simulink model "equal_area_piston_sfctrl"  (R2020a)
settings: Solver=ode23tb  StartTime=0.0  StopTime=400  MaxStep=tsample  RelTol=tsample
values from neighbouring files (symbols this model uses):
  A = [0 1; 0 0]    [control_design.m]
  B = [0 1]'    [control_design.m]
  C = [k 0]    [control_design.m]
  K = acker(A,B,poles)    [control_design.m]
  L = acker(A',C',pole_so)'    [control_design.m]
  N = -1/(C*inv(A-B*K)*B)    [control_design.m]
undefined symbols (not defined in the file or in its folder): uc_mac
libraries: fl_lib x21, nesl_utility x20, engine_speed_ctrl_lib x1, engine_OM471_lib x1, load_sensing_pump_lib x1, hydrostatic_fourway_valve_bichamber_piston_lib x1, pm_linear_actuator_lib x1
settings Model: Creator=dbagn  LastModifiedBy=dbagn
settings SolverCC: ZeroCrossControl=DisableAll
settings DataIOCC: SaveTime=off  ReturnWorkspaceOutputs=off

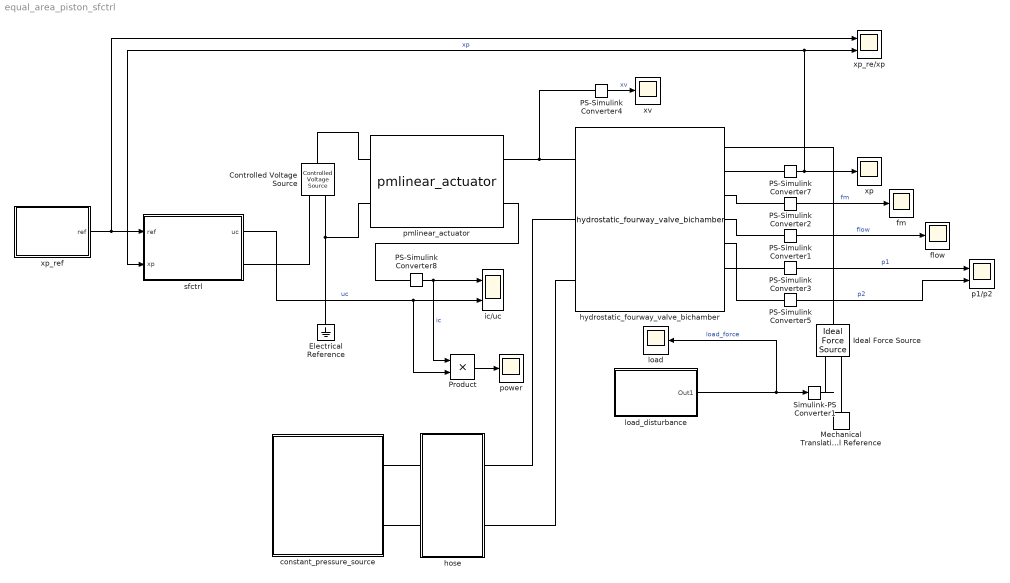
== system equal_area_piston_sfctrl ==
  Controlled Voltage Source : fl_lib/Electrical/Electrical Sources/Controlled Voltage Source
  Electrical Reference : fl_lib/Electrical/Electrical Elements/Electrical Reference
  Ideal Force Source : fl_lib/Mechanical/Mechanical Sources/Ideal Force Source
  Mechanical Translational Reference : fl_lib/Mechanical/Translational Elements/Mechanical Translational Reference
  PS-Simulink Converter{1..5,7..8} (7 alike) : nesl_utility/PS-Simulink Converter  PhysicalDomain=network_engine_domain  SubClassName=ps_output  LeftPortType=input  RightPortType=output  PseudoPeriodic=off  Frequencies=[]  Unit=inherit  AffineConversion=off
  Product : Product
  Simulink-PS Converter1 : nesl_utility/Simulink-PS Converter  PhysicalDomain=network_engine_domain  SubClassName=ps_input  LeftPortType=input  RightPortType=output  PseudoPeriodic=off  Frequencies=[]  NoiseDistribution=none  NoiseParameters=[]  Unit=N  AffineConversion=off  FilteringAndDerivatives=provide  SimscapeFilterOrder=1  InputFilterTimeConstant=0.001  UdotUserProvided=0
  constant_pressure_source : Subsystem
  flow : Scope
  fm : Scope
  hose : Subsystem
  hydrostatic_fourway_valve_bichamber : hydrostatic_fourway_valve_bichamber_piston_lib/hydrostatic_fourway_valve_bichamber  bulk=1.2e9 Pa  rho=850 kg/m^3  D1=0.1 m  D2=0.1 m  Lp=1 m  xv_max=2.75 mm  mp=25 kg  kp=1e5 N/m  bp=2e2 N/(m/s)  q1_specify=off  q1_priority=None  q1=0 m^3/s  q1_nominal_specify=off  q1_nominal_unit=m^3/s  q1_nominal_value=1  q2_specify=off  q2_priority=None  q2=0 m^3/s  q2_nominal_specify=off  q2_nominal_unit=m^3/s  q2_nominal_value=1  qin_specify=off  qin_priority=None  qin=0 m^3/s  qin_nominal_specify=off  qin_nominal_unit=m^3/s  qin_nominal_value=1  qout_specify=off  qout_priority=None  qout=0 m^3/s  qout_nominal_specify=off  qout_nominal_unit=m^3/s  qout_nominal_value=1  p1_specify=off  p1_priority=High  p1=25 bar  p1_nominal_specify=off  p1_nominal_unit=bar  p1_nominal_value=1  p2_specify=off  p2_priority=High  p2=25 bar  p2_nominal_specify=off  p2_nominal_unit=bar  p2_nominal_value=1  fp_specify=off  fp_priority=None  fp=0 N  fp_nominal_specify=off  fp_nominal_unit=N  fp_nominal_value=1  vp_specify=off  vp_priority=None  vp=0 m/s  vp_nominal_specify=off  vp_nominal_unit=m/s  vp_nominal_value=1  xp_specify=off  xp_priority=High  xp=500 mm  xp_nominal_specify=off  xp_nominal_unit=mm  xp_nominal_value=1
      settings: InternalSimscapePortConfiguration="{\"Bottom\":[],\"Left\":[{\"id\":\"xv\",\"label\":\"xv\",\"type\":\"input\"},{\"id\":\"S\",\"label\":\"S\",\"type\":\"foundation.hydraulic.hydraulic\"},{\"id\":\"T\",\"label\":\"T\",\"type\":\"foundation.hydraulic.hydraulic\"}],\"Right\":[{\"id\":\"P\",\"label\":\"P\",\"type\":\"foundation.mechanical.translational.translational\"},{\"id\":\"xp_out\",\"label\":\"xp\",\"type\":\"output\"},{\"id\":\"mforce\",\"label\":\"fm\",\"type\":\"output\"},{\"id\":\"q1_out\",\"label\":\"q1\",\"type\":\"output\"},{\"id\":\"q2_out\",\"label\":\"q2\",\"type\":\"output\"},{\"id\":\"p1_out\",\"label\":\"p1\",\"type\":\"output\"},{\"id\":\"p2_out\",\"label\":\"p2\",\"type\":\"output\"}],\"Top\":[]}"
  ic/uc : Scope  NumInputPorts=2
  load : Scope
  load_disturbance : Subsystem
  p1/p2 : Scope  NumInputPorts=2
  pmlinear_actuator : pm_linear_actuator_lib/pmlinear_actuator  Bm=1 s*V/m^2  mv=0.05 kg  Lc=0.01 H  Rc=10 Ohm  bv=2000 N/(m/s)  h=0.05 m  xv_max=2.75 mm  n=1000  uc_specify=off  uc_priority=None  uc=0 V  uc_nominal_specify=off  uc_nominal_unit=V  uc_nominal_value=1  ic_specify=off  ic_priority=High  ic=0 A  ic_nominal_specify=off  ic_nominal_unit=A  ic_nominal_value=1  vv_specify=off  vv_priority=None  vv=0 m/s  vv_nominal_specify=off  vv_nominal_unit=m/s  vv_nominal_value=1  xv_specify=off  xv_priority=None  xv=0 m  xv_nominal_specify=off  xv_nominal_unit=m  xv_nominal_value=1
      settings: InternalSimscapePortConfiguration="{\"Bottom\":[],\"Left\":[{\"id\":\"ucp\",\"label\":\"ucp\",\"type\":\"foundation.electrical.electrical\"},{\"id\":\"ucn\",\"label\":\"ucn\",\"type\":\"foundation.electrical.electrical\"}],\"Right\":[{\"id\":\"xv_out\",\"label\":\"xv\",\"type\":\"output\"},{\"id\":\"ic_out\",\"label\":\"ic\",\"type\":\"output\"}],\"Top\":[]}"
  power : Scope
  sfctrl : Subsystem
  xp : Scope
  xp_re/xp : Scope  NumInputPorts=2
  xp_ref : Subsystem
  xv : Scope
  wires:
  load_disturbance/1(Out1) -> load/1, Simulink-PS Converter1/1  "load_force"
  PS-Simulink Converter7/1 -> xp_re/xp/2, sfctrl/2(xp), xp/1  "xp"
  PS-Simulink Converter1/1 -> flow/1  "flow"
  PS-Simulink Converter2/1 -> fm/1  "fm"
  PS-Simulink Converter3/1 -> p1/p2/1  "p1"
  xp_ref/1(ref) -> xp_re/xp/1, sfctrl/1(ref)
  PS-Simulink Converter5/1 -> p1/p2/2  "p2"
  PS-Simulink Converter8/1 -> Product/1, ic/uc/1  "ic"
  sfctrl/1("uc ") -> Product/2, ic/uc/2  "uc"
  Product/1 -> power/1
  PS-Simulink Converter4/1 -> xv/1  "xv"
  connections:
  Mechanical Translational Reference/LConn1 -- Ideal Force Source/RConn2
  Simulink-PS Converter1/RConn1 -- Ideal Force Source/RConn1
  constant_pressure_source/RConn1 -- hose/LConn1
  constant_pressure_source/RConn2 -- hose/LConn2
  hydrostatic_fourway_valve_bichamber/LConn2 -- hose/RConn1
  hydrostatic_fourway_valve_bichamber/LConn3 -- hose/RConn2
  hydrostatic_fourway_valve_bichamber/RConn4 -- PS-Simulink Converter1/LConn1
  hydrostatic_fourway_valve_bichamber/RConn3 -- PS-Simulink Converter2/LConn1
  hydrostatic_fourway_valve_bichamber/RConn2 -- PS-Simulink Converter7/LConn1
  hydrostatic_fourway_valve_bichamber/RConn1 -- Ideal Force Source/LConn1
  hydrostatic_fourway_valve_bichamber/RConn5 -- PS-Simulink Converter3/LConn1
  hydrostatic_fourway_valve_bichamber/RConn6 -- PS-Simulink Converter5/LConn1
  Electrical Reference/LConn1 -- pmlinear_actuator/LConn2 -- Controlled Voltage Source/RConn2
  pmlinear_actuator/LConn1 -- Controlled Voltage Source/LConn1
  pmlinear_actuator/RConn1 -- PS-Simulink Converter4/LConn1 -- hydrostatic_fourway_valve_bichamber/LConn1
  pmlinear_actuator/RConn2 -- PS-Simulink Converter8/LConn1
  sfctrl/RConn1 -- Controlled Voltage Source/RConn1

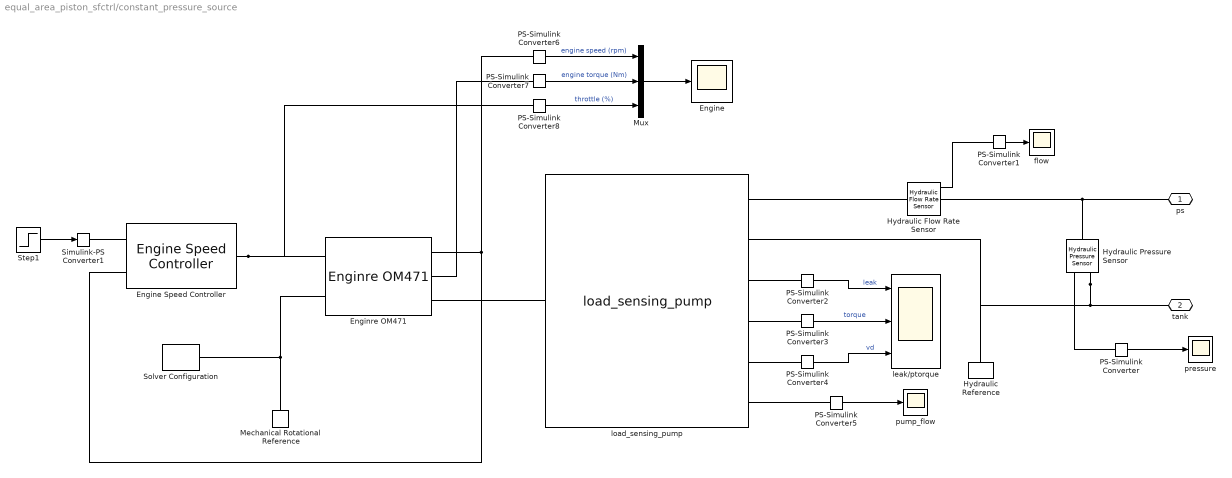
== system equal_area_piston_sfctrl/constant_pressure_source ==
  Engine : Scope
  Engine Speed Controller : engine_speed_ctrl_lib/Engine Speed Controller  kp=1e-3/2 s  kint=1e-2/2  kd=0 s^2  t_out_specify=off  t_out_priority=High  t_out=0  t_out_nominal_specify=off  t_out_nominal_unit=1  t_out_nominal_value=1
      settings: InternalSimscapePortConfiguration="{\"Bottom\":[],\"Left\":[{\"id\":\"we_ref\",\"label\":\"we_ref\",\"type\":\"input\"},{\"id\":\"we\",\"label\":\"we\",\"type\":\"input\"}],\"Right\":[{\"id\":\"theta\",\"label\":\"theta\",\"type\":\"output\"}],\"Top\":[]}"
  Enginre OM471 : engine_OM471_lib/Enginre OM471  dynamic_responce=simscape.enum.onoff.on  cshaft_inertia=5 kg*m^2  initial_speed=800
      settings: InternalSimscapePortConfiguration="{\"Bottom\":[],\"Left\":[{\"id\":\"theta\",\"label\":\"theta\",\"type\":\"input\"},{\"id\":\"C\",\"label\":\"C\",\"type\":\"foundation.mechanical.rotational.rotational\"}],\"Right\":[{\"id\":\"we\",\"label\":\"we\",\"type\":\"output\"},{\"id\":\"te\",\"label\":\"te\",\"type\":\"output\"},{\"id\":\"D\",\"label\":\"D\",\"type\":\"foundation.mechanical.rotational.rotational\"}],\"Top\":[]}"
  Hydraulic Flow Rate Sensor : fl_lib/Hydraulic/Hydraulic Sensors/Hydraulic Flow Rate Sensor
  Hydraulic Pressure Sensor : fl_lib/Hydraulic/Hydraulic Sensors/Hydraulic Pressure Sensor
  Hydraulic Reference : fl_lib/Hydraulic/Hydraulic Elements/Hydraulic Reference
  Mechanical Rotational Reference : fl_lib/Mechanical/Rotational Elements/Mechanical Rotational Reference
  Mux : Mux  Inputs=3
  PS-Simulink Converter : nesl_utility/PS-Simulink Converter  PhysicalDomain=network_engine_domain  SubClassName=ps_output  LeftPortType=input  RightPortType=output  PseudoPeriodic=off  Frequencies=[]  Unit=bar  AffineConversion=on
  PS-Simulink Converter1 : nesl_utility/PS-Simulink Converter  PhysicalDomain=network_engine_domain  SubClassName=ps_output  LeftPortType=input  RightPortType=output  PseudoPeriodic=off  Frequencies=[]  Unit=l/min  AffineConversion=on
  PS-Simulink Converter{2..5} (4 alike) : nesl_utility/PS-Simulink Converter  PhysicalDomain=network_engine_domain  SubClassName=ps_output  LeftPortType=input  RightPortType=output  PseudoPeriodic=off  Frequencies=[]  Unit=1  AffineConversion=off
  PS-Simulink Converter6 : nesl_utility/PS-Simulink Converter  PhysicalDomain=network_engine_domain  SubClassName=ps_output  LeftPortType=input  RightPortType=output  PseudoPeriodic=off  Frequencies=[]  Unit=inherit  AffineConversion=off
  PS-Simulink Converter7 : nesl_utility/PS-Simulink Converter  PhysicalDomain=network_engine_domain  SubClassName=ps_output  LeftPortType=input  RightPortType=output  PseudoPeriodic=off  Frequencies=[]  Unit=inherit  AffineConversion=off
  PS-Simulink Converter8 : nesl_utility/PS-Simulink Converter  PhysicalDomain=network_engine_domain  SubClassName=ps_output  LeftPortType=input  RightPortType=output  PseudoPeriodic=off  Frequencies=[]  Unit=inherit  AffineConversion=off
  Simulink-PS Converter1 : nesl_utility/Simulink-PS Converter  PhysicalDomain=network_engine_domain  SubClassName=ps_input  LeftPortType=input  RightPortType=output  PseudoPeriodic=off  Frequencies=[]  NoiseDistribution=none  NoiseParameters=[]  Unit=rpm  AffineConversion=off  FilteringAndDerivatives=filter  SimscapeFilterOrder=2  InputFilterTimeConstant=0.1  UdotUserProvided=0
  Solver Configuration : nesl_utility/Solver Configuration  PhysicalDomain=network_engine_domain  SubClassName=solver  LeftPortType=input  RightPortType=generic  Tones=[]  Harmonics=[]  SimulateNoise=off  Profile=off  UseLocalSampling=off  EnableSwitchedLinearOptims=on  FrequencyDomain=off  UseCCode=off  RelTol=0.001  AbsTol=1e-06  MinStep=1e-09  ToWorkspace=off  RevertToSquareIcSolve=off  NumHomotopyIterations=100  PhasorMode=off  PhasorModeNumHarmonics=1  DoDC=off  ResidualTolerance=1e-09  UseLocalSolver=on  LocalSolverChoice=NE_BACKWARD_EULER_ADVANCER  LocalSolverSampleTime=tsample  DoFixedCost=on  MaxNonlinIter=3  MaxModeIter=2  LinearAlgebra=auto  EquationFormulation=NE_TIME_EF  DelaysMemoryBudget=1024  AutomaticFiltering=on  FilteringTimeConstant=tsample  PartitionStorageMethod=AS_NEEDED  PartitionMemoryBudget=1024  PartitionMethod=ROBUST
  Step1 : Step  Time=0  After=1900  SampleTime=0
  flow : Scope
  leak/ptorque : Scope  NumInputPorts=3
  load_sensing_pump : load_sensing_pump_lib/load_sensing_pump  vd_lim_max=0.98  vd_lim_min=-0.98  Vd_nom=62.3 cm^3/rev  dp_ref=250 bar  kpc=8  kic=8 1/s  p_set=250 bar  p_reg=8 bar  x_rv_max=32 mm  te_specify=off  te_priority=None  te=0 N*m  te_nominal_specify=off  te_nominal_unit=N*m  te_nominal_value=1  qA_specify=off  qA_priority=None  qA=0 m^3/s  qA_nominal_specify=off  qA_nominal_unit=m^3/s  qA_nominal_value=1  qB_specify=off  qB_priority=None  qB=0 m^3/s  qB_nominal_specify=off  qB_nominal_unit=m^3/s  qB_nominal_value=1  qd_specify=off  qd_priority=None  qd=0 m^3/s  qd_nominal_specify=off  qd_nominal_unit=m^3/s  qd_nominal_value=1  dp_specify=off  dp_priority=None  dp=0 Pa  dp_nominal_specify=off  dp_nominal_unit=Pa  dp_nominal_value=1  vd_specify=on  vd_priority=High  vd=0  vd_nominal_specify=off  vd_nominal_unit=1  vd_nominal_value=1  vd_i_specify=off  vd_i_priority=None  vd_i=0  vd_i_nominal_specify=off  vd_i_nominal_unit=1  vd_i_nominal_value=1  we_specify=off  we_priority=None  we=0 rad/s  we_nominal_specify=off  we_nominal_unit=rad/s  we_nominal_value=1
      settings: InternalSimscapePortConfiguration="{\"Bottom\":[],\"Left\":[{\"id\":\"cW\",\"label\":\"cW\",\"type\":\"foundation.mechanical.rotational.rotational\"}],\"Right\":[{\"id\":\"cA\",\"label\":\"cA\",\"type\":\"foundation.hydraulic.hydraulic\"},{\"id\":\"cB\",\"label\":\"cB\",\"type\":\"foundation.hydraulic.hydraulic\"},{\"id\":\"qr\",\"label\":\"qr\",\"type\":\"output\"},{\"id\":\"tm\",\"label\":\"tm\",\"type\":\"output\"},{\"id\":\"vdi\",\"label\":\"vdi\",\"type\":\"output\"},{\"id\":\"pflow\",\"label\":\"pflow\",\"type\":\"output\"}],\"Top\":[]}"
  pressure : Scope
  pump_flow : Scope
  ps : PMIOPort  Side=Right
  tank : PMIOPort  Port=2  Side=Right
  wires:
  PS-Simulink Converter2/1 -> leak/ptorque/1  "leak"
  PS-Simulink Converter/1 -> pressure/1
  PS-Simulink Converter5/1 -> pump_flow/1
  PS-Simulink Converter1/1 -> flow/1
  PS-Simulink Converter3/1 -> leak/ptorque/2  "torque"
  PS-Simulink Converter4/1 -> leak/ptorque/3  "vd"
  Step1/1 -> Simulink-PS Converter1/1
  PS-Simulink Converter6/1 -> Mux/1  "engine speed (rpm)"
  PS-Simulink Converter7/1 -> Mux/2  "engine torque (Nm)"
  Mux/1 -> Engine/1
  PS-Simulink Converter8/1 -> Mux/3  "throttle (%)"
  connections:
  PS-Simulink Converter/LConn1 -- Hydraulic Pressure Sensor/RConn2
  Hydraulic Flow Rate Sensor/RConn2 -- ps/RConn1 -- Hydraulic Pressure Sensor/LConn1
  load_sensing_pump/RConn6 -- PS-Simulink Converter5/LConn1
  load_sensing_pump/RConn5 -- PS-Simulink Converter4/LConn1
  PS-Simulink Converter3/LConn1 -- load_sensing_pump/RConn4
  Hydraulic Flow Rate Sensor/RConn1 -- PS-Simulink Converter1/LConn1
  Hydraulic Flow Rate Sensor/LConn1 -- load_sensing_pump/RConn1
  load_sensing_pump/RConn3 -- PS-Simulink Converter2/LConn1
  Enginre OM471/RConn3 -- load_sensing_pump/LConn1
  Enginre OM471/RConn1 -- Engine Speed Controller/LConn2 -- PS-Simulink Converter6/LConn1
  Engine Speed Controller/LConn1 -- Simulink-PS Converter1/RConn1
  Hydraulic Pressure Sensor/RConn1 -- load_sensing_pump/RConn2 -- Hydraulic Reference/LConn1 -- tank/RConn1
  Engine Speed Controller/RConn1 -- Enginre OM471/LConn1 -- PS-Simulink Converter8/LConn1
  Mechanical Rotational Reference/LConn1 -- Enginre OM471/LConn2 -- Solver Configuration/RConn1
  Enginre OM471/RConn2 -- PS-Simulink Converter7/LConn1

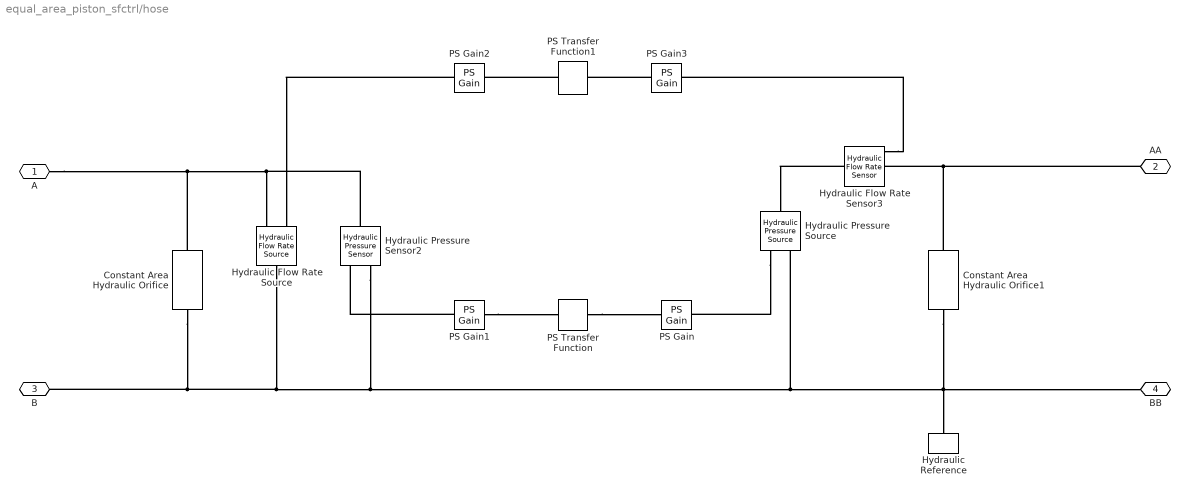
== system equal_area_piston_sfctrl/hose ==
  Constant Area Hydraulic Orifice : fl_lib/Hydraulic/Hydraulic Elements/Constant Area Hydraulic Orifice  area=1e-8 m^2  C_d=0.7  lam_spec=1  B_lam=0.999  Re_cr=12  q_specify=off  q_priority=None  q=0.001 m^3/s  q_nominal_specify=off  q_nominal_unit=m^3/s  q_nominal_value=1  p_specify=off  p_priority=None  p=0 Pa  p_nominal_specify=off  p_nominal_unit=Pa  p_nominal_value=1
      settings: SourceProductBaseCode=SS  InternalSimscapePortConfiguration="{\"Bottom\":[],\"Left\":[{\"id\":\"A\",\"label\":\"A\",\"type\":\"foundation.hydraulic.hydraulic\"}],\"Right\":[{\"id\":\"B\",\"label\":\"B\",\"type\":\"foundation.hydraulic.hydraulic\"}],\"Top\":[]}"
  Constant Area Hydraulic Orifice1 : fl_lib/Hydraulic/Hydraulic Elements/Constant Area Hydraulic Orifice  area=1e-8 m^2  C_d=0.7  lam_spec=1  B_lam=0.999  Re_cr=12  q_specify=off  q_priority=None  q=0.001 m^3/s  q_nominal_specify=off  q_nominal_unit=m^3/s  q_nominal_value=1  p_specify=off  p_priority=None  p=0 Pa  p_nominal_specify=off  p_nominal_unit=Pa  p_nominal_value=1
      settings: SourceProductBaseCode=SS  InternalSimscapePortConfiguration="{\"Bottom\":[],\"Left\":[{\"id\":\"A\",\"label\":\"A\",\"type\":\"foundation.hydraulic.hydraulic\"}],\"Right\":[{\"id\":\"B\",\"label\":\"B\",\"type\":\"foundation.hydraulic.hydraulic\"}],\"Top\":[]}"
  Hydraulic Flow Rate Sensor3 : fl_lib/Hydraulic/Hydraulic Sensors/Hydraulic Flow Rate Sensor
  Hydraulic Flow Rate Source : fl_lib/Hydraulic/Hydraulic Sources/Hydraulic Flow Rate Source
      settings: SourceProductBaseCode=SS  InternalSimscapePortConfiguration="{\"Bottom\":[],\"Left\":[{\"id\":\"P\",\"label\":\"P\",\"type\":\"foundation.hydraulic.hydraulic\"}],\"Right\":[{\"id\":\"S\",\"label\":\"S\",\"type\":\"input\"},{\"id\":\"T\",\"label\":\"T\",\"type\":\"foundation.hydraulic.hydraulic\"}],\"Top\":[]}"
  Hydraulic Pressure Sensor2 : fl_lib/Hydraulic/Hydraulic Sensors/Hydraulic Pressure Sensor
  Hydraulic Pressure Source : fl_lib/Hydraulic/Hydraulic Sources/Hydraulic Pressure Source
      settings: SourceProductBaseCode=SS  InternalSimscapePortConfiguration="{\"Bottom\":[],\"Left\":[{\"id\":\"P\",\"label\":\"P\",\"type\":\"foundation.hydraulic.hydraulic\"}],\"Right\":[{\"id\":\"S\",\"label\":\"S\",\"type\":\"input\"},{\"id\":\"T\",\"label\":\"T\",\"type\":\"foundation.hydraulic.hydraulic\"}],\"Top\":[]}"
  Hydraulic Reference : fl_lib/Hydraulic/Hydraulic Elements/Hydraulic Reference
  PS Gain : fl_lib/Physical Signals/Functions/PS Gain  gain=1 Pa
  PS Gain1 : fl_lib/Physical Signals/Functions/PS Gain  gain=1 Pa^-1
  PS Gain2 : fl_lib/Physical Signals/Functions/PS Gain  gain=1 m^3/s
  PS Gain3 : fl_lib/Physical Signals/Functions/PS Gain  gain=1 m^-3*s
  PS Transfer Function : fl_lib/Physical Signals/Linear Operators/PS Transfer Function  transfer_function_type=foundation.enum.transfer_function_type.lag  T=0.1 s  T1=2 s  T2=1 s  y0=0
      settings: SourceProductBaseCode=SS  InternalSimscapePortConfiguration="{\"Bottom\":[],\"Left\":[{\"id\":\"U\",\"label\":\"\",\"type\":\"input\"}],\"Right\":[{\"id\":\"Y\",\"label\":\"\",\"type\":\"output\"}],\"Top\":[]}"
  PS Transfer Function1 : fl_lib/Physical Signals/Linear Operators/PS Transfer Function  transfer_function_type=foundation.enum.transfer_function_type.lag  T=0.1 s  T1=2 s  T2=1 s  y0=0
      settings: SourceProductBaseCode=SS  InternalSimscapePortConfiguration="{\"Bottom\":[],\"Left\":[{\"id\":\"U\",\"label\":\"\",\"type\":\"input\"}],\"Right\":[{\"id\":\"Y\",\"label\":\"\",\"type\":\"output\"}],\"Top\":[]}"
  A : PMIOPort  Side=Left
  AA : PMIOPort  Port=2  Side=Right
  B : PMIOPort  Port=3  Side=Left
  BB : PMIOPort  Port=4  Side=Right
  connections:
  AA/RConn1 -- Constant Area Hydraulic Orifice1/LConn1 -- Hydraulic Flow Rate Sensor3/RConn2
  PS Gain2/RConn1 -- Hydraulic Flow Rate Source/RConn1
  Hydraulic Flow Rate Sensor3/RConn1 -- PS Gain3/LConn1
  Hydraulic Flow Rate Sensor3/LConn1 -- Hydraulic Pressure Source/LConn1
  Hydraulic Pressure Source/RConn1 -- PS Gain/RConn1
  PS Gain1/LConn1 -- Hydraulic Pressure Sensor2/RConn2
  Hydraulic Pressure Source/RConn2 -- Hydraulic Pressure Sensor2/RConn1 -- Constant Area Hydraulic Orifice/RConn1 -- B/RConn1 -- Hydraulic Flow Rate Source/LConn1 -- Constant Area Hydraulic Orifice1/RConn1 -- Hydraulic Reference/LConn1 -- BB/RConn1
  PS Transfer Function1/RConn1 -- PS Gain2/LConn1
  PS Transfer Function/RConn1 -- PS Gain/LConn1
  A/RConn1 -- Constant Area Hydraulic Orifice/LConn1 -- Hydraulic Pressure Sensor2/LConn1 -- Hydraulic Flow Rate Source/RConn2
  PS Gain3/RConn1 -- PS Transfer Function1/LConn1
  PS Gain1/RConn1 -- PS Transfer Function/LConn1

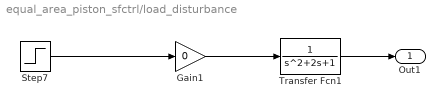
== system equal_area_piston_sfctrl/load_disturbance ==
  Gain1 : Gain  Gain=0
  Step7 : Step  Time=5  After=12500  SampleTime=0
  Transfer Fcn1 : TransferFcn
  Out1 : Outport
  wires:
  Gain1/1 -> Transfer Fcn1/1
  Transfer Fcn1/1 -> Out1/1
  Step7/1 -> Gain1/1

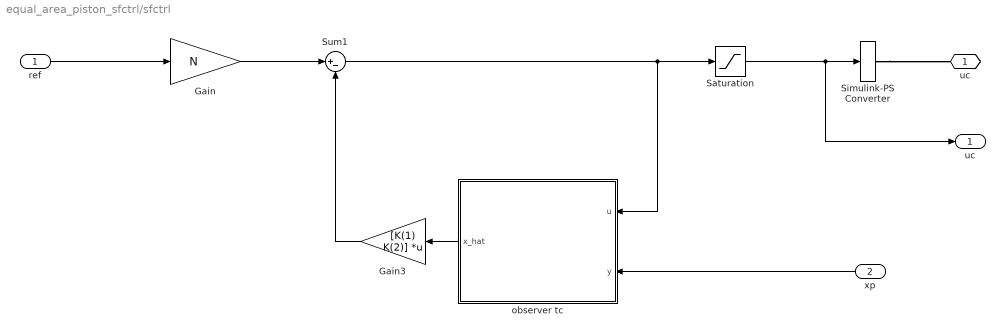
== system equal_area_piston_sfctrl/sfctrl ==
  ref : Inport
  xp : Inport  Port=2
  Gain : Gain  Gain=N
  Gain3 : Gain  Gain=[K(1) K(2)]  Multiplication=Matrix(K*u)
  Saturation : Saturate  UpperLimit=uc_mac  LowerLimit=-uc_mac
  Simulink-PS Converter : nesl_utility/Simulink-PS Converter  PhysicalDomain=network_engine_domain  SubClassName=ps_input  LeftPortType=input  RightPortType=output  PseudoPeriodic=off  Frequencies=[]  NoiseDistribution=none  NoiseParameters=[]  Unit=V  AffineConversion=off  FilteringAndDerivatives=provide  SimscapeFilterOrder=1  InputFilterTimeConstant=0.001  UdotUserProvided=0
  Sum1 : Sum  Inputs=|+-
  observer tc : Subsystem
  uc : PMIOPort  Side=Right
  "uc " : Outport
  wires:
  observer tc/1(x_hat) -> Gain3/1
  Gain/1 -> Sum1/1
  Gain3/1 -> Sum1/2
  Sum1/1 -> observer tc/1(u), Saturation/1
  xp/1 -> observer tc/2(y)
  ref/1 -> Gain/1
  Saturation/1 -> "uc "/1, Simulink-PS Converter/1
  connections:
  Simulink-PS Converter/RConn1 -- uc/RConn1

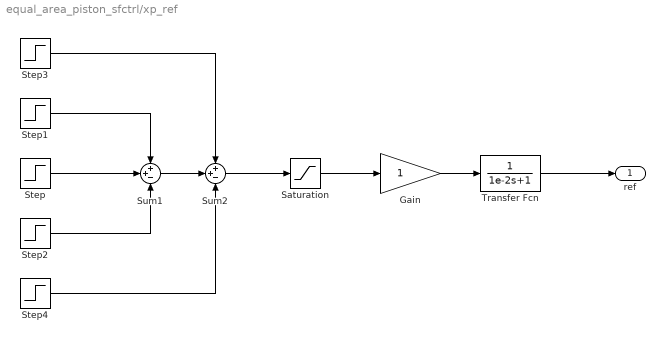
== system equal_area_piston_sfctrl/xp_ref ==
  Gain : Gain
  Saturation : Saturate  UpperLimit=1.1  LowerLimit=-1.1
  Step : Step  Time=50  After=0.5  SampleTime=0
  Step1 : Step  Time=80  SampleTime=0
  Step2 : Step  Time=120  After=2.6  SampleTime=0
  Step3 : Step  Time=150  After=1.4  SampleTime=0
  Step4 : Step  Time=180  After=0.1  SampleTime=0
  Sum1 : Sum  Inputs=++-
  Sum2 : Sum  Inputs=++-
  Transfer Fcn : TransferFcn  Denominator=[1e-2 1]
  ref : Outport
  wires:
  Step/1 -> Sum1/2
  Gain/1 -> Transfer Fcn/1
  Transfer Fcn/1 -> ref/1
  Step1/1 -> Sum1/1
  Step2/1 -> Sum1/3
  Sum1/1 -> Sum2/2
  Step3/1 -> Sum2/1
  Step4/1 -> Sum2/3
  Sum2/1 -> Saturation/1
  Saturation/1 -> Gain/1

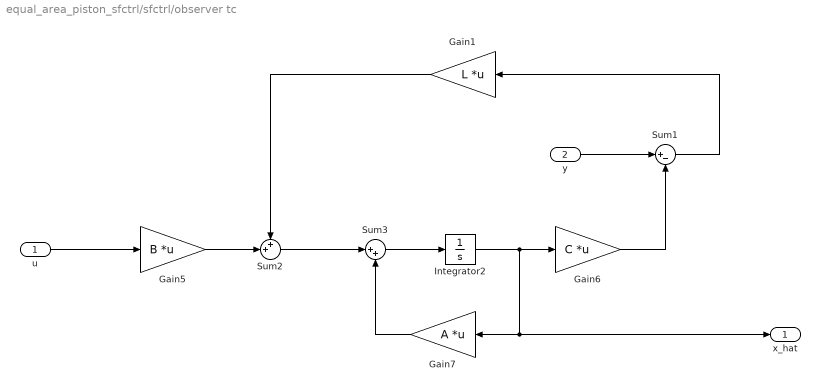
== system equal_area_piston_sfctrl/sfctrl/observer tc ==
  u : Inport
  y : Inport  Port=2
  Gain1 : Gain  Gain=L  Multiplication=Matrix(K*u)
  Gain5 : Gain  Gain=B  Multiplication=Matrix(K*u)
  Gain6 : Gain  Gain=C  Multiplication=Matrix(K*u)
  Gain7 : Gain  Gain=A  Multiplication=Matrix(K*u)
  Integrator2 : Integrator
  Sum1 : Sum  Inputs=|+-
  Sum2 : Sum  Inputs=++|
  Sum3 : Sum  Inputs=|++
  x_hat : Outport
  wires:
  Sum2/1 -> Sum3/1
  Integrator2/1 -> x_hat/1, Gain7/1, Gain6/1
  Sum3/1 -> Integrator2/1
  Gain7/1 -> Sum3/2
  y/1 -> Sum1/1
  Gain6/1 -> Sum1/2
  Sum1/1 -> Gain1/1
  u/1 -> Gain5/1
  Gain1/1 -> Sum2/1
  Gain5/1 -> Sum2/2
